simulink model "niof_model"  (R2021a)
settings: Solver=ode23tb  StartTime=0.0  StopTime=2  RelTol=1e-3
values from neighbouring files (symbols this model uses):
  h0 = ds.DateTime(1).Hour + ds.DateTime(1).Minute/60    [compiler_niof_model.m]
  S_area_hole = 0.01    [set_params_blocks.m]
undefined symbols (not defined in the file or in its folder): crop_GH1_NFT_slot1___C, crop_GH1_NFT_slot1___N, crop_GH1_NFT_slot1___R, crop_GH1_NFT_slot2___C, crop_GH1_NFT_slot2___N, crop_GH1_NFT_slot2___R, crop_GH1_NFT_slot3___C, crop_GH1_NFT_slot3___N, crop_GH1_NFT_slot3___R, crop_GH1_NFT_slot4___C, crop_GH1_NFT_slot4___N, crop_GH1_NFT_slot4___R, crop_GH1_RF_slot1___C, crop_GH1_RF_slot1___N, crop_GH1_RF_slot1___R, crop_GH1_RF_slot2___C, crop_GH1_RF_slot2___N, crop_GH1_RF_slot2___R, crop_GH1_RF_slot3___C, crop_GH1_RF_slot3___N, crop_GH1_RF_slot3___R, crop_GH1_RF_slot4___C, crop_GH1_RF_slot4___N, crop_GH1_RF_slot4___R, crop_GH2_RF_slot1___C, crop_GH2_RF_slot1___N, crop_GH2_RF_slot1___R, crop_GH2_RF_slot2___C, crop_GH2_RF_slot2___N, crop_GH2_RF_slot2___R, crop_GH2_RF_slot3___C, crop_GH2_RF_slot3___N, crop_GH2_RF_slot3___R, crop_GH2_RF_slot4___C, crop_GH2_RF_slot4___N, crop_GH2_RF_slot4___R, crop_GH2_TRAD_slot1___C, crop_GH2_TRAD_slot1___N, crop_GH2_TRAD_slot1___R, crop_GH2_TRAD_slot2___C, crop_GH2_TRAD_slot2___N, crop_GH2_TRAD_slot2___R, crop_GH2_TRAD_slot3___C, crop_GH2_TRAD_slot3___N, crop_GH2_TRAD_slot3___R, crop_GH2_TRAD_slot4___C, crop_GH2_TRAD_slot4___N, crop_GH2_TRAD_slot4___R, fish, GH3_Tank1_tend, GH3_Tank2_tend, GH3_Tank3_tend, GH3_Tank4_tend, tp_biofilter___T, tp_fish_C___T, tp_fish_M___T, tp_fish_S___T, tp_fish_T___T, tp_GH1_bio___T, tp_GH1_NFT___T ... (+3)
libraries: HORTISIM x152
(part 4 of 4)

== system niof_model/GH2/TRAD System/Subsystem1/TankToCrop Parser Several ==
  note: $m^3/s$
  C1 : Inport
  C2 : Inport  Port=2
  C3 : Inport  Port=3
  C4 : Inport  Port=4
  WT : Inport  Port=5
  Bus Selector1 : BusSelector  OutputSignals=R_uptake,Fout
  Gain : Gain  Gain=-1
  Selector : Selector  InputPortWidth=4  IndexOptions=Index vector (dialog)  Indices=[1]  OutputSizes=1
  Selector1 : Selector  InputPortWidth=4  IndexOptions=Index vector (dialog)  Indices=[2]  OutputSizes=1
  Selector2 : Selector  NumberOfDimensions=2  InputPortWidth=2  IndexOptions=Select all,Index vector (dialog)  Indices=[1],1  OutputSizes=1,1
  Selector3 : Selector  NumberOfDimensions=2  InputPortWidth=2  IndexOptions=Select all,Index vector (dialog)  Indices=[2],2  OutputSizes=1,1
  Selector4 : Selector  InputPortWidth=4  IndexOptions=Index vector (dialog)  Indices=[3]  OutputSizes=1
  Selector5 : Selector  InputPortWidth=4  IndexOptions=Index vector (dialog)  Indices=[4]  OutputSizes=1
  Selector6 : Selector  NumberOfDimensions=2  InputPortWidth=2  IndexOptions=Select all,Index vector (dialog)  Indices=[2],3  OutputSizes=1,1
  Selector7 : Selector  NumberOfDimensions=2  InputPortWidth=2  IndexOptions=Select all,Index vector (dialog)  Indices=[2],4  OutputSizes=1,1
  Subsystem : Subsystem
  Subsystem1 : Subsystem
  Subsystem2 : Subsystem
  Subsystem3 : Subsystem
  Out Bus Element : Outport  PortName=Subs1  Element=uptake.Nutrients
  Out Bus Element1 : Outport  PortName=Subs1  Element=Uptake.Water
  Out Bus Element2 : Outport  Port=2  PortName=Subs2  Element=Uptake.Nutrients
  Out Bus Element3 : Outport  Port=2  PortName=Subs2  Element=Uptake.Water
  Out Bus Element6 : Outport  Port=3  PortName=Subs3  Element=Uptake.Nutrients
  Out Bus Element4 : Outport  Port=3  PortName=Subs3  Element=Uptake.Water
  Out Bus Element7 : Outport  Port=4  PortName=Subs4  Element=Uptake.Nutrients
  Out Bus Element5 : Outport  Port=4  PortName=Subs4  Element=Uptake.Water
  wires:
  WT/1 -> Bus Selector1/1
  Bus Selector1/1 -> Gain/1  "<R_uptake>"
  Gain/1 -> Selector7/1, Selector6/1, Selector3/1, Selector2/1  "<Demand>"
  Selector2/1 -> Out Bus Element/1
  Selector3/1 -> Out Bus Element2/1
  Selector/1 -> Subsystem/1(In1)
  C1/1 -> Subsystem/2(In2)
  Subsystem/1(Out1) -> Out Bus Element1/1
  Selector1/1 -> Subsystem1/1(In1)
  C2/1 -> Subsystem1/2(C2)
  Subsystem1/1(Out1) -> Out Bus Element3/1
  Selector4/1 -> Subsystem2/1(In1)
  C3/1 -> Subsystem2/2(C2)
  Bus Selector1/2 -> Selector5/1, Selector4/1, Selector1/1, Selector/1  "<Fout>"
  Selector5/1 -> Subsystem3/1(In1)
  C4/1 -> Subsystem3/2(C2)
  Subsystem2/1("Subs3 ") -> Out Bus Element4/1
  Subsystem3/1(Subs4) -> Out Bus Element5/1
  Selector6/1 -> Out Bus Element6/1
  Selector7/1 -> Out Bus Element7/1

== system niof_model/GH1/NFT System/Reorder signals/Subsystem1/Crop Interactio with Climate ==
  C1 : Inport
  C2 : Inport  Port=2
  C3 : Inport  Port=3
  C4 : Inport  Port=4
  Crop2ExtArray{,1..3} (4 alike) : HORTISIM/Other  Functions/Crop2ExtArray  SystemSampleTime=-1  VariantActivationTime=update diagram  Latency=0  AutoFrameSizeCalculation=off
      settings: SourceProductName=Horti Simulator
  Demux : Demux
  Sum : Sum  Inputs=+  CollapseMode=Specified dimension  CollapseDim=2
  Vector Concatenate : Concatenate  NumInputs=4  Mode=Multidimensional array  ConcatenateDimension=2
  Out Bus Element : Outport  PortName=OutBus  Element=HeatVars.QV
  Out Bus Element1 : Outport  PortName=OutBus  Element=HeatVars.QT
  Out Bus Element2 : Outport  PortName=OutBus  Element=A_v
  Out Bus Element3 : Outport  PortName=OutBus  Element=CC
  wires:
  C1/1 -> Crop2ExtArray/1
  C2/1 -> Crop2ExtArray1/1
  C3/1 -> Crop2ExtArray2/1
  C4/1 -> Crop2ExtArray3/1
  Crop2ExtArray3/1 -> Vector Concatenate/4
  Crop2ExtArray2/1 -> Vector Concatenate/3
  Crop2ExtArray1/1 -> Vector Concatenate/2
  Crop2ExtArray/1 -> Vector Concatenate/1
  Vector Concatenate/1 -> Sum/1
  Sum/1 -> Demux/1
  Demux/1 -> Out Bus Element/1
  Demux/2 -> Out Bus Element1/1
  Demux/3 -> Out Bus Element2/1
  Demux/4 -> Out Bus Element3/1

== system niof_model/GH1/NFT System/Reorder signals/Subsystem1/TankToCrop Parser Several ==
  note: $m^3/s$
  C1 : Inport
  C2 : Inport  Port=2
  C3 : Inport  Port=3
  C4 : Inport  Port=4
  WT : Inport  Port=5
  Bus Selector1 : BusSelector  OutputSignals=R_uptake,Fout
  Gain : Gain  Gain=-1
  Selector : Selector  InputPortWidth=4  IndexOptions=Index vector (dialog)  Indices=[1]  OutputSizes=1
  Selector1 : Selector  InputPortWidth=4  IndexOptions=Index vector (dialog)  Indices=[2]  OutputSizes=1
  Selector2 : Selector  NumberOfDimensions=2  InputPortWidth=2  IndexOptions=Select all,Index vector (dialog)  Indices=[1],1  OutputSizes=1,1
  Selector3 : Selector  NumberOfDimensions=2  InputPortWidth=2  IndexOptions=Select all,Index vector (dialog)  Indices=[2],2  OutputSizes=1,1
  Selector4 : Selector  InputPortWidth=4  IndexOptions=Index vector (dialog)  Indices=[3]  OutputSizes=1
  Selector5 : Selector  InputPortWidth=4  IndexOptions=Index vector (dialog)  Indices=[4]  OutputSizes=1
  Selector6 : Selector  NumberOfDimensions=2  InputPortWidth=2  IndexOptions=Select all,Index vector (dialog)  Indices=[2],3  OutputSizes=1,1
  Selector7 : Selector  NumberOfDimensions=2  InputPortWidth=2  IndexOptions=Select all,Index vector (dialog)  Indices=[2],4  OutputSizes=1,1
  Subsystem : Subsystem
  Subsystem1 : Subsystem
  Subsystem2 : Subsystem
  Subsystem3 : Subsystem
  Out Bus Element : Outport  PortName=Subs1  Element=Uptake.Nutrients
  Out Bus Element1 : Outport  PortName=Subs1  Element=Uptake.Water
  Out Bus Element2 : Outport  Port=2  PortName=Subs2  Element=Uptake.Nutrients
  Out Bus Element3 : Outport  Port=2  PortName=Subs2  Element=Uptake.Water
  Out Bus Element6 : Outport  Port=3  PortName=Subs3  Element=Uptake.Nutrients
  Out Bus Element4 : Outport  Port=3  PortName=Subs3  Element=Uptake.Water
  Out Bus Element7 : Outport  Port=4  PortName=Subs4  Element=Uptake.Nutrients
  Out Bus Element5 : Outport  Port=4  PortName=Subs4  Element=Uptake.Water
  wires:
  WT/1 -> Bus Selector1/1
  Bus Selector1/1 -> Gain/1  "<R_uptake>"
  Gain/1 -> Selector7/1, Selector6/1, Selector3/1, Selector2/1  "<Demand>"
  Selector2/1 -> Out Bus Element/1
  Selector3/1 -> Out Bus Element2/1
  Selector/1 -> Subsystem/1(In1)
  C1/1 -> Subsystem/2(In2)
  Subsystem/1(Out1) -> Out Bus Element1/1
  Selector1/1 -> Subsystem1/1(In1)
  C2/1 -> Subsystem1/2(C2)
  Subsystem1/1(Out1) -> Out Bus Element3/1
  Selector4/1 -> Subsystem2/1(In1)
  C3/1 -> Subsystem2/2(C2)
  Bus Selector1/2 -> Selector5/1, Selector4/1, Selector1/1, Selector/1  "<Fout>"
  Selector5/1 -> Subsystem3/1(In1)
  C4/1 -> Subsystem3/2(C2)
  Subsystem2/1("Subs3 ") -> Out Bus Element4/1
  Subsystem3/1(Subs4) -> Out Bus Element5/1
  Selector6/1 -> Out Bus Element6/1
  Selector7/1 -> Out Bus Element7/1

== system niof_model/GH1/RF System/Subsystem1/TankToCrop Parser Several/Subsystem ==
  note: $kg\{H_2O\}/s$
  In1 : Inport
  In2 : Inport  Port=2
  Bus Selector : BusSelector  OutputSignals=f
  Bus Selector2 : BusSelector  OutputSignals=A_v
  Divide : Product  Inputs=*/
  Water Density [kg/m^3] : Gain  Gain=997
  Out1 : Outport
  wires:
  In2/1 -> Bus Selector2/1
  Water Density [kg/m^3]/1 -> Divide/1
  In1/1 -> Bus Selector/1
  Bus Selector/1 -> Water Density [kg/m^3]/1  "<f>"
  Divide/1 -> Out1/1
  Bus Selector2/1 -> Divide/2  "<A_v>"

== system niof_model/GH1/RF System/Subsystem1/TankToCrop Parser Several/Subsystem1 ==
  note: $kg\{H_2O\}/s$
  In1 : Inport
  C2 : Inport  Port=2
  Bus Selector3 : BusSelector  OutputSignals=A_v
  Bus Selector4 : BusSelector  OutputSignals=f
  Divide1 : Product  Inputs=*/
  Water Density [kg/m^3]1 : Gain  Gain=997
  Out1 : Outport
  wires:
  In1/1 -> Bus Selector4/1
  Water Density [kg/m^3]1/1 -> Divide1/1
  Bus Selector4/1 -> Water Density [kg/m^3]1/1  "<f>"
  Divide1/1 -> Out1/1
  Bus Selector3/1 -> Divide1/2  "<A_v>"
  C2/1 -> Bus Selector3/1

== system niof_model/GH1/RF System/Subsystem1/TankToCrop Parser Several/Subsystem2 ==
  note: $kg\{H_2O\}/s$
  In1 : Inport
  C2 : Inport  Port=2
  Bus Selector3 : BusSelector  OutputSignals=A_v
  Bus Selector4 : BusSelector  OutputSignals=f
  Divide1 : Product  Inputs=*/
  Water Density [kg/m^3]1 : Gain  Gain=997
  "Subs3 " : Outport
  wires:
  In1/1 -> Bus Selector4/1
  Water Density [kg/m^3]1/1 -> Divide1/1
  Bus Selector4/1 -> Water Density [kg/m^3]1/1  "<f>"
  Divide1/1 -> "Subs3 "/1
  Bus Selector3/1 -> Divide1/2  "<A_v>"
  C2/1 -> Bus Selector3/1

== system niof_model/GH1/RF System/Subsystem1/TankToCrop Parser Several/Subsystem3 ==
  note: $kg\{H_2O\}/s$
  In1 : Inport
  C2 : Inport  Port=2
  Bus Selector3 : BusSelector  OutputSignals=A_v
  Bus Selector4 : BusSelector  OutputSignals=f
  Divide1 : Product  Inputs=*/
  Water Density [kg/m^3]1 : Gain  Gain=997
  Subs4 : Outport
  wires:
  In1/1 -> Bus Selector4/1
  Water Density [kg/m^3]1/1 -> Divide1/1
  Bus Selector4/1 -> Water Density [kg/m^3]1/1  "<f>"
  Divide1/1 -> Subs4/1
  Bus Selector3/1 -> Divide1/2  "<A_v>"
  C2/1 -> Bus Selector3/1

== system niof_model/GH2/RF System/Subsystem1/TankToCrop Parser Several/Subsystem ==
  note: $kg\{H_2O\}/s$
  In1 : Inport
  In2 : Inport  Port=2
  Bus Selector : BusSelector  OutputSignals=f
  Bus Selector2 : BusSelector  OutputSignals=A_v
  Divide : Product  Inputs=*/
  Water Density [kg/m^3] : Gain  Gain=997
  Out1 : Outport
  wires:
  In2/1 -> Bus Selector2/1
  Water Density [kg/m^3]/1 -> Divide/1
  In1/1 -> Bus Selector/1
  Bus Selector/1 -> Water Density [kg/m^3]/1  "<f>"
  Divide/1 -> Out1/1
  Bus Selector2/1 -> Divide/2  "<A_v>"

== system niof_model/GH2/RF System/Subsystem1/TankToCrop Parser Several/Subsystem1 ==
  note: $kg\{H_2O\}/s$
  In1 : Inport
  C2 : Inport  Port=2
  Bus Selector3 : BusSelector  OutputSignals=A_v
  Bus Selector4 : BusSelector  OutputSignals=f
  Divide1 : Product  Inputs=*/
  Water Density [kg/m^3]1 : Gain  Gain=997
  Out1 : Outport
  wires:
  In1/1 -> Bus Selector4/1
  Water Density [kg/m^3]1/1 -> Divide1/1
  Bus Selector4/1 -> Water Density [kg/m^3]1/1  "<f>"
  Divide1/1 -> Out1/1
  Bus Selector3/1 -> Divide1/2  "<A_v>"
  C2/1 -> Bus Selector3/1

== system niof_model/GH2/RF System/Subsystem1/TankToCrop Parser Several/Subsystem2 ==
  note: $kg\{H_2O\}/s$
  In1 : Inport
  C2 : Inport  Port=2
  Bus Selector3 : BusSelector  OutputSignals=A_v
  Bus Selector4 : BusSelector  OutputSignals=f
  Divide1 : Product  Inputs=*/
  Water Density [kg/m^3]1 : Gain  Gain=997
  "Subs3 " : Outport
  wires:
  In1/1 -> Bus Selector4/1
  Water Density [kg/m^3]1/1 -> Divide1/1
  Bus Selector4/1 -> Water Density [kg/m^3]1/1  "<f>"
  Divide1/1 -> "Subs3 "/1
  Bus Selector3/1 -> Divide1/2  "<A_v>"
  C2/1 -> Bus Selector3/1

== system niof_model/GH2/RF System/Subsystem1/TankToCrop Parser Several/Subsystem3 ==
  note: $kg\{H_2O\}/s$
  In1 : Inport
  C2 : Inport  Port=2
  Bus Selector3 : BusSelector  OutputSignals=A_v
  Bus Selector4 : BusSelector  OutputSignals=f
  Divide1 : Product  Inputs=*/
  Water Density [kg/m^3]1 : Gain  Gain=997
  Subs4 : Outport
  wires:
  In1/1 -> Bus Selector4/1
  Water Density [kg/m^3]1/1 -> Divide1/1
  Bus Selector4/1 -> Water Density [kg/m^3]1/1  "<f>"
  Divide1/1 -> Subs4/1
  Bus Selector3/1 -> Divide1/2  "<A_v>"
  C2/1 -> Bus Selector3/1

== system niof_model/GH2/TRAD System/Subsystem1/TankToCrop Parser Several/Subsystem ==
  note: $kg\{H_2O\}/s$
  In1 : Inport
  In2 : Inport  Port=2
  Bus Selector : BusSelector  OutputSignals=f
  Bus Selector2 : BusSelector  OutputSignals=A_v
  Divide : Product  Inputs=*/
  Water Density [kg/m^3] : Gain  Gain=997
  Out1 : Outport
  wires:
  In2/1 -> Bus Selector2/1
  Water Density [kg/m^3]/1 -> Divide/1
  In1/1 -> Bus Selector/1
  Bus Selector/1 -> Water Density [kg/m^3]/1  "<f>"
  Divide/1 -> Out1/1
  Bus Selector2/1 -> Divide/2  "<A_v>"

== system niof_model/GH2/TRAD System/Subsystem1/TankToCrop Parser Several/Subsystem1 ==
  note: $kg\{H_2O\}/s$
  In1 : Inport
  C2 : Inport  Port=2
  Bus Selector3 : BusSelector  OutputSignals=A_v
  Bus Selector4 : BusSelector  OutputSignals=f
  Divide1 : Product  Inputs=*/
  Water Density [kg/m^3]1 : Gain  Gain=997
  Out1 : Outport
  wires:
  In1/1 -> Bus Selector4/1
  Water Density [kg/m^3]1/1 -> Divide1/1
  Bus Selector4/1 -> Water Density [kg/m^3]1/1  "<f>"
  Divide1/1 -> Out1/1
  Bus Selector3/1 -> Divide1/2  "<A_v>"
  C2/1 -> Bus Selector3/1

== system niof_model/GH2/TRAD System/Subsystem1/TankToCrop Parser Several/Subsystem2 ==
  note: $kg\{H_2O\}/s$
  In1 : Inport
  C2 : Inport  Port=2
  Bus Selector3 : BusSelector  OutputSignals=A_v
  Bus Selector4 : BusSelector  OutputSignals=f
  Divide1 : Product  Inputs=*/
  Water Density [kg/m^3]1 : Gain  Gain=997
  "Subs3 " : Outport
  wires:
  In1/1 -> Bus Selector4/1
  Water Density [kg/m^3]1/1 -> Divide1/1
  Bus Selector4/1 -> Water Density [kg/m^3]1/1  "<f>"
  Divide1/1 -> "Subs3 "/1
  Bus Selector3/1 -> Divide1/2  "<A_v>"
  C2/1 -> Bus Selector3/1

== system niof_model/GH2/TRAD System/Subsystem1/TankToCrop Parser Several/Subsystem3 ==
  note: $kg\{H_2O\}/s$
  In1 : Inport
  C2 : Inport  Port=2
  Bus Selector3 : BusSelector  OutputSignals=A_v
  Bus Selector4 : BusSelector  OutputSignals=f
  Divide1 : Product  Inputs=*/
  Water Density [kg/m^3]1 : Gain  Gain=997
  Subs4 : Outport
  wires:
  In1/1 -> Bus Selector4/1
  Water Density [kg/m^3]1/1 -> Divide1/1
  Bus Selector4/1 -> Water Density [kg/m^3]1/1  "<f>"
  Divide1/1 -> Subs4/1
  Bus Selector3/1 -> Divide1/2  "<A_v>"
  C2/1 -> Bus Selector3/1

== system niof_model/GH1/NFT System/Reorder signals/Subsystem1/TankToCrop Parser Several/Subsystem ==
  note: $kg\{H_2O\}/s$
  In1 : Inport
  In2 : Inport  Port=2
  Bus Selector : BusSelector  OutputSignals=f
  Bus Selector2 : BusSelector  OutputSignals=A_v
  Divide : Product  Inputs=*/
  Water Density [kg/m^3] : Gain  Gain=997
  Out1 : Outport
  wires:
  In2/1 -> Bus Selector2/1
  Water Density [kg/m^3]/1 -> Divide/1
  In1/1 -> Bus Selector/1
  Bus Selector/1 -> Water Density [kg/m^3]/1  "<f>"
  Divide/1 -> Out1/1
  Bus Selector2/1 -> Divide/2  "<A_v>"

== system niof_model/GH1/NFT System/Reorder signals/Subsystem1/TankToCrop Parser Several/Subsystem1 ==
  note: $kg\{H_2O\}/s$
  In1 : Inport
  C2 : Inport  Port=2
  Bus Selector3 : BusSelector  OutputSignals=A_v
  Bus Selector4 : BusSelector  OutputSignals=f
  Divide1 : Product  Inputs=*/
  Water Density [kg/m^3]1 : Gain  Gain=997
  Out1 : Outport
  wires:
  In1/1 -> Bus Selector4/1
  Water Density [kg/m^3]1/1 -> Divide1/1
  Bus Selector4/1 -> Water Density [kg/m^3]1/1  "<f>"
  Divide1/1 -> Out1/1
  Bus Selector3/1 -> Divide1/2  "<A_v>"
  C2/1 -> Bus Selector3/1

== system niof_model/GH1/NFT System/Reorder signals/Subsystem1/TankToCrop Parser Several/Subsystem2 ==
  note: $kg\{H_2O\}/s$
  In1 : Inport
  C2 : Inport  Port=2
  Bus Selector3 : BusSelector  OutputSignals=A_v
  Bus Selector4 : BusSelector  OutputSignals=f
  Divide1 : Product  Inputs=*/
  Water Density [kg/m^3]1 : Gain  Gain=997
  "Subs3 " : Outport
  wires:
  In1/1 -> Bus Selector4/1
  Water Density [kg/m^3]1/1 -> Divide1/1
  Bus Selector4/1 -> Water Density [kg/m^3]1/1  "<f>"
  Divide1/1 -> "Subs3 "/1
  Bus Selector3/1 -> Divide1/2  "<A_v>"
  C2/1 -> Bus Selector3/1

== system niof_model/GH1/NFT System/Reorder signals/Subsystem1/TankToCrop Parser Several/Subsystem3 ==
  note: $kg\{H_2O\}/s$
  In1 : Inport
  C2 : Inport  Port=2
  Bus Selector3 : BusSelector  OutputSignals=A_v
  Bus Selector4 : BusSelector  OutputSignals=f
  Divide1 : Product  Inputs=*/
  Water Density [kg/m^3]1 : Gain  Gain=997
  Subs4 : Outport
  wires:
  In1/1 -> Bus Selector4/1
  Water Density [kg/m^3]1/1 -> Divide1/1
  Bus Selector4/1 -> Water Density [kg/m^3]1/1  "<f>"
  Divide1/1 -> Subs4/1
  Bus Selector3/1 -> Divide1/2  "<A_v>"
  C2/1 -> Bus Selector3/1
